simulink model "PWMGenerator"  (R2014a)
settings: Solver=FixedStepDiscrete  StartTime=0.0  StopTime=500000  FixedStep=1  RelTol=1e-3
libraries: hdlsllib x15
settings Model: Creator=rogers.a  LastModifiedBy=rogers.a
settings OptimizationCC: BlockReduction=off  ConditionallyExecuteInputs=off  InlineParams=on
settings DebuggingCC: AlgebraicLoopMsg=error
settings HardwareCC: ProdHWDeviceType=ASIC/FPGA->ASIC/FPGA  ProdEqTarget=off

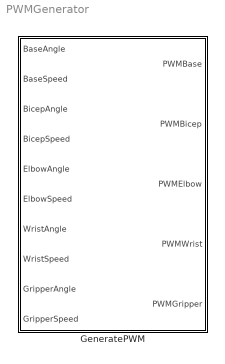
== system PWMGenerator ==
  GeneratePWM : Subsystem  TreatAsAtomicUnit=on

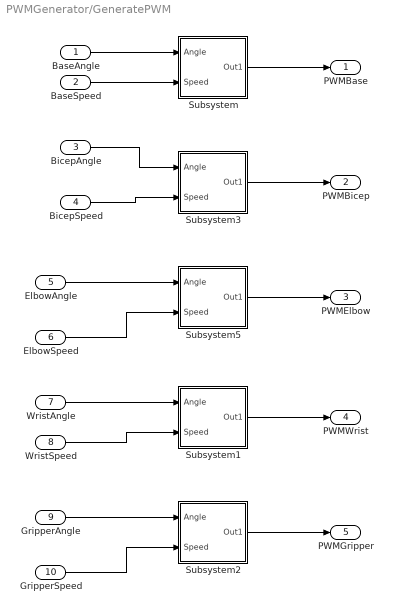
== system PWMGenerator/GeneratePWM ==
  "BaseAngle " : Inport  OutDataTypeStr=int8
  "BaseSpeed " : Inport  Port=2  OutDataTypeStr=int8
  BicepAngle : Inport  Port=3  OutDataTypeStr=int8
  "BicepSpeed " : Inport  Port=4  OutDataTypeStr=int8
  ElbowAngle : Inport  Port=5  OutDataTypeStr=int8
  "ElbowSpeed " : Inport  Port=6  OutDataTypeStr=int8
  WristAngle : Inport  Port=7  OutDataTypeStr=int8
  WristSpeed : Inport  Port=8  OutDataTypeStr=int8
  "GripperAngle " : Inport  Port=9  OutDataTypeStr=int8
  GripperSpeed : Inport  Port=10  OutDataTypeStr=int8
  Subsystem : Subsystem
  Subsystem1 : Subsystem
  Subsystem2 : Subsystem
  Subsystem3 : Subsystem
  Subsystem5 : Subsystem
  PWMBase : Outport
  PWMBicep : Outport  Port=2
  PWMElbow : Outport  Port=3
  PWMWrist : Outport  Port=4
  PWMGripper : Outport  Port=5
  wires:
  Subsystem3/1(Out1) -> PWMBicep/1
  Subsystem5/1(Out1) -> PWMElbow/1
  ElbowAngle/1 -> Subsystem5/1(Angle)
  "ElbowSpeed "/1 -> Subsystem5/2("Speed ")
  Subsystem/1(Out1) -> PWMBase/1
  Subsystem1/1(Out1) -> PWMWrist/1
  WristAngle/1 -> Subsystem1/1(Angle)
  WristSpeed/1 -> Subsystem1/2("Speed ")
  "BaseSpeed "/1 -> Subsystem/2("Speed ")
  "BicepSpeed "/1 -> Subsystem3/2("Speed ")
  "BaseAngle "/1 -> Subsystem/1(Angle)
  BicepAngle/1 -> Subsystem3/1(Angle)
  GripperSpeed/1 -> Subsystem2/2("Speed ")
  "GripperAngle "/1 -> Subsystem2/1(Angle)
  Subsystem2/1(Out1) -> PWMGripper/1

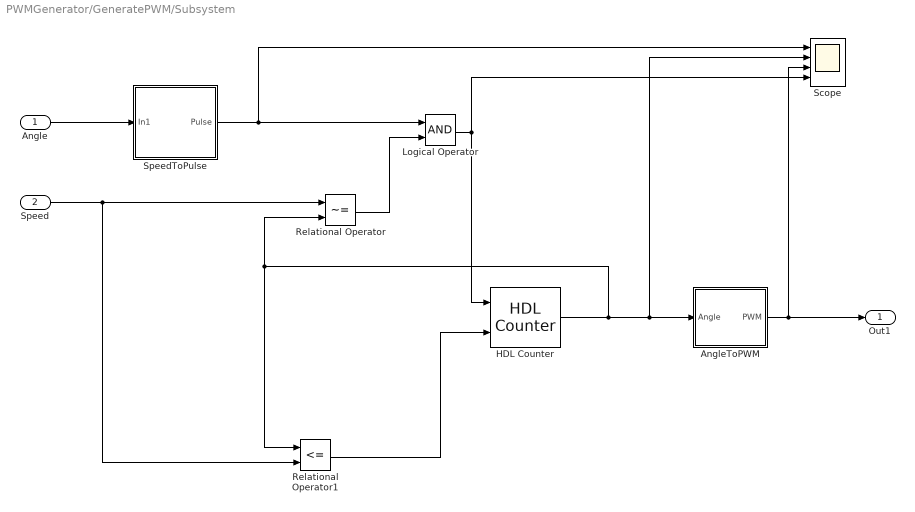
== system PWMGenerator/GeneratePWM/Subsystem ==
  Angle : Inport
  "Speed " : Inport  Port=2
  "AngleToPWM " : Subsystem
  HDL Counter : hdlsllib/HDL Operations/HDL Counter  CountType=Count limited  CountInit=0  CountStep=1  CountMax=180  CountFromType=Specify  CountFrom=0  CountResetPort=off  CountLoadPort=off  CountEnbPort=on  CountDirPort=on  CountDataType=Unsigned  CountWordLen=8  CountFracLen=0  CountSampTime=1
  Logical Operator : Logic  AllPortsSameDT=off  OutDataTypeStr=boolean
  Relational Operator : RelationalOperator  Operator=~=  OutDataTypeStr=boolean
  Relational Operator1 : RelationalOperator  Operator=<=  OutDataTypeStr=boolean
  Scope : Scope  NumInputPorts=4
      settings: YMin=0~0~0~0  YMax=1~300~1~1
  SpeedToPulse : Subsystem
  Out1 : Outport  OutDataTypeStr=boolean
  wires:
  "AngleToPWM "/1("PWM ") -> Scope/3, Out1/1
  HDL Counter/1 -> "AngleToPWM "/1("Angle "), Scope/2, Relational Operator1/1, Relational Operator/2
  Relational Operator1/1 -> HDL Counter/2
  Logical Operator/1 -> Scope/4, HDL Counter/1
  Relational Operator/1 -> Logical Operator/2
  "Speed "/1 -> Relational Operator/1, Relational Operator1/2
  SpeedToPulse/1(Pulse) -> Scope/1, Logical Operator/1
  Angle/1 -> SpeedToPulse/1(In1)

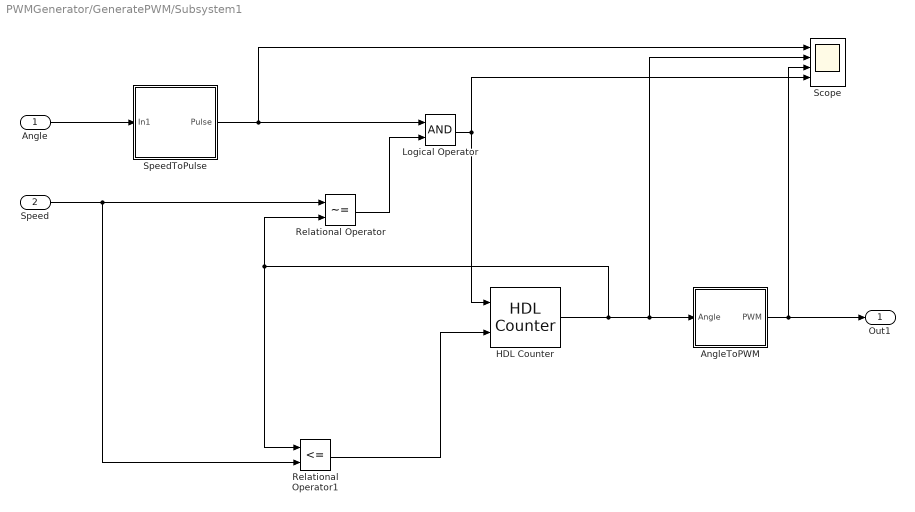
== system PWMGenerator/GeneratePWM/Subsystem1 ==
  Angle : Inport
  "Speed " : Inport  Port=2
  "AngleToPWM " : Subsystem
  HDL Counter : hdlsllib/HDL Operations/HDL Counter  CountType=Count limited  CountInit=0  CountStep=1  CountMax=180  CountFromType=Specify  CountFrom=0  CountResetPort=off  CountLoadPort=off  CountEnbPort=on  CountDirPort=on  CountDataType=Unsigned  CountWordLen=8  CountFracLen=0  CountSampTime=1
  Logical Operator : Logic  AllPortsSameDT=off  OutDataTypeStr=boolean
  Relational Operator : RelationalOperator  Operator=~=  OutDataTypeStr=boolean
  Relational Operator1 : RelationalOperator  Operator=<=  OutDataTypeStr=boolean
  Scope : Scope  NumInputPorts=4
      settings: YMin=0~0~0~0  YMax=1~300~1~1
  SpeedToPulse : Subsystem
  Out1 : Outport  OutDataTypeStr=boolean
  wires:
  "AngleToPWM "/1("PWM ") -> Scope/3, Out1/1
  HDL Counter/1 -> "AngleToPWM "/1("Angle "), Scope/2, Relational Operator1/1, Relational Operator/2
  Relational Operator1/1 -> HDL Counter/2
  Logical Operator/1 -> Scope/4, HDL Counter/1
  Relational Operator/1 -> Logical Operator/2
  "Speed "/1 -> Relational Operator/1, Relational Operator1/2
  SpeedToPulse/1(Pulse) -> Scope/1, Logical Operator/1
  Angle/1 -> SpeedToPulse/1(In1)

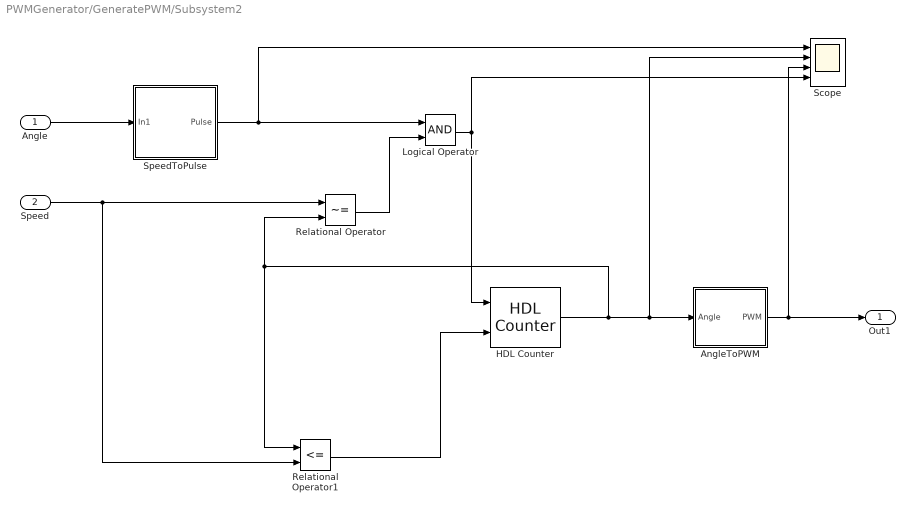
== system PWMGenerator/GeneratePWM/Subsystem2 ==
  Angle : Inport
  "Speed " : Inport  Port=2
  "AngleToPWM " : Subsystem
  HDL Counter : hdlsllib/HDL Operations/HDL Counter  CountType=Count limited  CountInit=0  CountStep=1  CountMax=180  CountFromType=Specify  CountFrom=0  CountResetPort=off  CountLoadPort=off  CountEnbPort=on  CountDirPort=on  CountDataType=Unsigned  CountWordLen=8  CountFracLen=0  CountSampTime=1
  Logical Operator : Logic  AllPortsSameDT=off  OutDataTypeStr=boolean
  Relational Operator : RelationalOperator  Operator=~=  OutDataTypeStr=boolean
  Relational Operator1 : RelationalOperator  Operator=<=  OutDataTypeStr=boolean
  Scope : Scope  NumInputPorts=4
      settings: YMin=0~0~0~0  YMax=1~300~1~1
  SpeedToPulse : Subsystem
  Out1 : Outport  OutDataTypeStr=boolean
  wires:
  "AngleToPWM "/1("PWM ") -> Scope/3, Out1/1
  HDL Counter/1 -> "AngleToPWM "/1("Angle "), Scope/2, Relational Operator1/1, Relational Operator/2
  Relational Operator1/1 -> HDL Counter/2
  Logical Operator/1 -> Scope/4, HDL Counter/1
  Relational Operator/1 -> Logical Operator/2
  "Speed "/1 -> Relational Operator/1, Relational Operator1/2
  SpeedToPulse/1(Pulse) -> Scope/1, Logical Operator/1
  Angle/1 -> SpeedToPulse/1(In1)

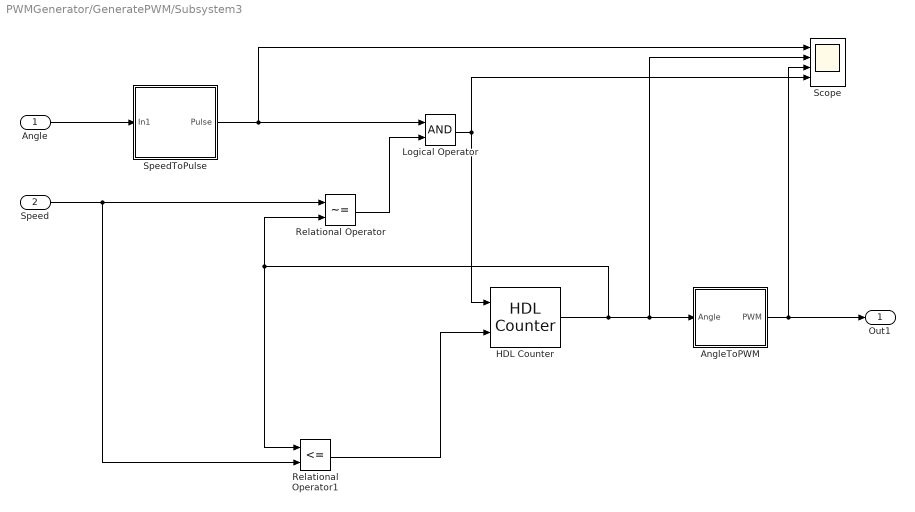
== system PWMGenerator/GeneratePWM/Subsystem3 ==
  Angle : Inport
  "Speed " : Inport  Port=2
  "AngleToPWM " : Subsystem
  HDL Counter : hdlsllib/HDL Operations/HDL Counter  CountType=Count limited  CountInit=0  CountStep=1  CountMax=180  CountFromType=Specify  CountFrom=0  CountResetPort=off  CountLoadPort=off  CountEnbPort=on  CountDirPort=on  CountDataType=Unsigned  CountWordLen=8  CountFracLen=0  CountSampTime=1
  Logical Operator : Logic  AllPortsSameDT=off  OutDataTypeStr=boolean
  Relational Operator : RelationalOperator  Operator=~=  OutDataTypeStr=boolean
  Relational Operator1 : RelationalOperator  Operator=<=  OutDataTypeStr=boolean
  Scope : Scope  NumInputPorts=4
      settings: YMin=0~0~0~0  YMax=1~300~1~1
  SpeedToPulse : Subsystem
  Out1 : Outport  OutDataTypeStr=boolean
  wires:
  "AngleToPWM "/1("PWM ") -> Scope/3, Out1/1
  HDL Counter/1 -> "AngleToPWM "/1("Angle "), Scope/2, Relational Operator1/1, Relational Operator/2
  Relational Operator1/1 -> HDL Counter/2
  Logical Operator/1 -> Scope/4, HDL Counter/1
  Relational Operator/1 -> Logical Operator/2
  "Speed "/1 -> Relational Operator/1, Relational Operator1/2
  SpeedToPulse/1(Pulse) -> Scope/1, Logical Operator/1
  Angle/1 -> SpeedToPulse/1(In1)

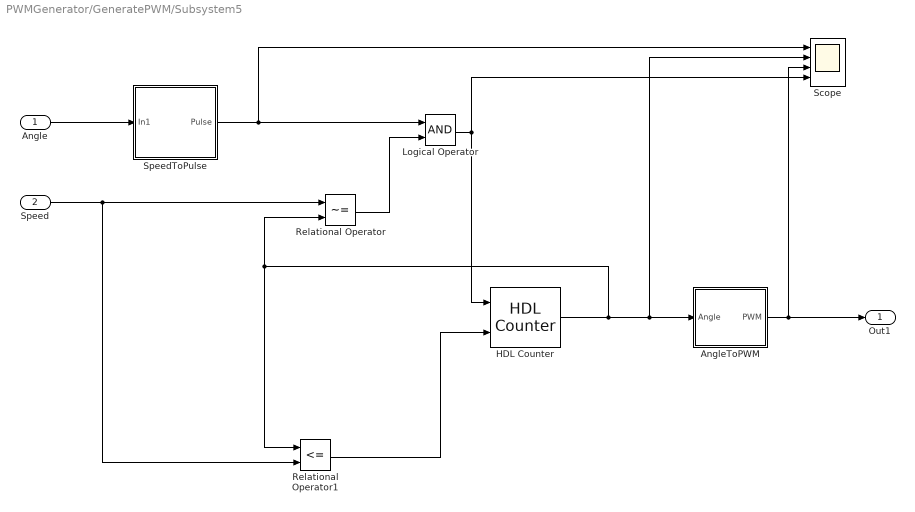
== system PWMGenerator/GeneratePWM/Subsystem5 ==
  Angle : Inport
  "Speed " : Inport  Port=2
  "AngleToPWM " : Subsystem
  HDL Counter : hdlsllib/HDL Operations/HDL Counter  CountType=Count limited  CountInit=0  CountStep=1  CountMax=180  CountFromType=Specify  CountFrom=0  CountResetPort=off  CountLoadPort=off  CountEnbPort=on  CountDirPort=on  CountDataType=Unsigned  CountWordLen=8  CountFracLen=0  CountSampTime=1
  Logical Operator : Logic  AllPortsSameDT=off  OutDataTypeStr=boolean
  Relational Operator : RelationalOperator  Operator=~=  OutDataTypeStr=boolean
  Relational Operator1 : RelationalOperator  Operator=<=  OutDataTypeStr=boolean
  Scope : Scope  NumInputPorts=4
      settings: YMin=0~0~0~0  YMax=1~300~1~1
  SpeedToPulse : Subsystem
  Out1 : Outport  OutDataTypeStr=boolean
  wires:
  "AngleToPWM "/1("PWM ") -> Scope/3, Out1/1
  HDL Counter/1 -> "AngleToPWM "/1("Angle "), Scope/2, Relational Operator1/1, Relational Operator/2
  Relational Operator1/1 -> HDL Counter/2
  Logical Operator/1 -> Scope/4, HDL Counter/1
  Relational Operator/1 -> Logical Operator/2
  "Speed "/1 -> Relational Operator/1, Relational Operator1/2
  SpeedToPulse/1(Pulse) -> Scope/1, Logical Operator/1
  Angle/1 -> SpeedToPulse/1(In1)

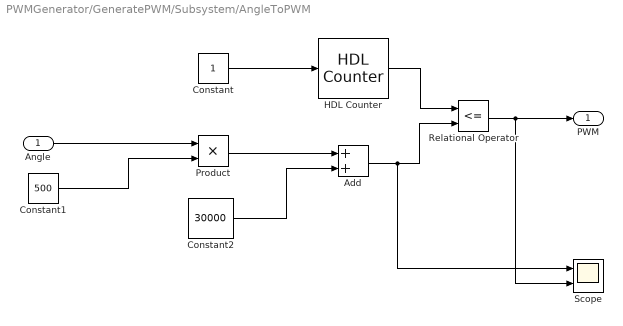
== system PWMGenerator/GeneratePWM/Subsystem/AngleToPWM  ==
  "Angle " : Inport  OutDataTypeStr=uint8
  Add : Sum
  Constant : Constant  OutDataTypeStr=boolean
  Constant1 : Constant  Value=500  OutDataTypeStr=uint32
  Constant2 : Constant  Value=30000  OutDataTypeStr=uint32
  HDL Counter : hdlsllib/HDL Operations/HDL Counter  CountType=Count limited  CountInit=0  CountStep=1  CountMax=1000000  CountFromType=Initial value  CountFrom=0  CountResetPort=off  CountLoadPort=off  CountEnbPort=on  CountDirPort=off  CountDataType=Unsigned  CountWordLen=32  CountFracLen=0  CountSampTime=1
  Product : Product  OutDataTypeStr=Inherit: Inherit via back propagation  SaturateOnIntegerOverflow=on
  Relational Operator : RelationalOperator  Operator=<=  OutDataTypeStr=boolean
  Scope : Scope  NumInputPorts=2
      settings: YMin=45000~-5  YMax=45000~5
  "PWM " : Outport
  wires:
  Add/1 -> Relational Operator/2, Scope/1
  Relational Operator/1 -> "PWM "/1, Scope/2
  "Angle "/1 -> Product/1
  Product/1 -> Add/1
  Constant1/1 -> Product/2
  Constant/1 -> HDL Counter/1
  Constant2/1 -> Add/2
  HDL Counter/1 -> Relational Operator/1

== system PWMGenerator/GeneratePWM/Subsystem/SpeedToPulse ==
  In1 : Inport
  Constant : Constant  Value=50000000  OutDataTypeStr=int32
  Constant1 : Constant  OutDataTypeStr=boolean
  Divide : Product  Inputs=*/  SaturateOnIntegerOverflow=on  RndMeth=Zero
  HDL Counter : hdlsllib/HDL Operations/HDL Counter  CountType=Free running  CountInit=0  CountStep=1  CountMax=10000  CountFromType=Initial value  CountFrom=0  CountResetPort=on  CountLoadPort=off  CountEnbPort=on  CountDirPort=off  CountDataType=Unsigned  CountWordLen=32  CountFracLen=0  CountSampTime=1
  Relational Operator : RelationalOperator  OutDataTypeStr=boolean
  Scope : Scope
  Pulse : Outport
  wires:
  Constant1/1 -> HDL Counter/2
  Relational Operator/1 -> HDL Counter/1, Scope/1, Pulse/1
  In1/1 -> Divide/2
  Divide/1 -> Relational Operator/2
  Constant/1 -> Divide/1
  HDL Counter/1 -> Relational Operator/1

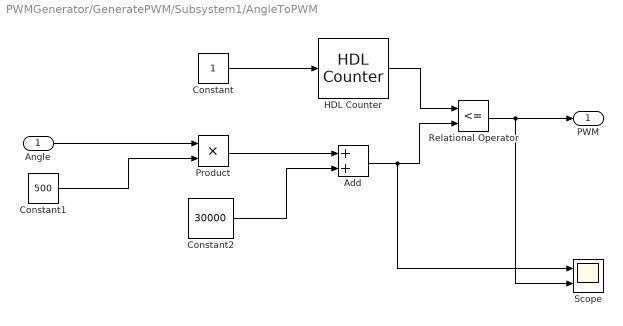
== system PWMGenerator/GeneratePWM/Subsystem1/AngleToPWM  ==
  "Angle " : Inport  OutDataTypeStr=uint8
  Add : Sum
  Constant : Constant  OutDataTypeStr=boolean
  Constant1 : Constant  Value=500  OutDataTypeStr=uint32
  Constant2 : Constant  Value=30000  OutDataTypeStr=uint32
  HDL Counter : hdlsllib/HDL Operations/HDL Counter  CountType=Count limited  CountInit=0  CountStep=1  CountMax=1000000  CountFromType=Initial value  CountFrom=0  CountResetPort=off  CountLoadPort=off  CountEnbPort=on  CountDirPort=off  CountDataType=Unsigned  CountWordLen=32  CountFracLen=0  CountSampTime=1
  Product : Product  OutDataTypeStr=Inherit: Inherit via back propagation  SaturateOnIntegerOverflow=on
  Relational Operator : RelationalOperator  Operator=<=  OutDataTypeStr=boolean
  Scope : Scope  NumInputPorts=2
      settings: YMin=45000~-5  YMax=45000~5
  "PWM " : Outport
  wires:
  Add/1 -> Relational Operator/2, Scope/1
  Relational Operator/1 -> "PWM "/1, Scope/2
  "Angle "/1 -> Product/1
  Product/1 -> Add/1
  Constant1/1 -> Product/2
  Constant/1 -> HDL Counter/1
  Constant2/1 -> Add/2
  HDL Counter/1 -> Relational Operator/1

== system PWMGenerator/GeneratePWM/Subsystem1/SpeedToPulse ==
  In1 : Inport
  Constant : Constant  Value=50000000  OutDataTypeStr=int32
  Constant1 : Constant  OutDataTypeStr=boolean
  Divide : Product  Inputs=*/  SaturateOnIntegerOverflow=on  RndMeth=Zero
  HDL Counter : hdlsllib/HDL Operations/HDL Counter  CountType=Free running  CountInit=0  CountStep=1  CountMax=10000  CountFromType=Initial value  CountFrom=0  CountResetPort=on  CountLoadPort=off  CountEnbPort=on  CountDirPort=off  CountDataType=Unsigned  CountWordLen=32  CountFracLen=0  CountSampTime=1
  Relational Operator : RelationalOperator  OutDataTypeStr=boolean
  Scope : Scope
  Pulse : Outport
  wires:
  Constant1/1 -> HDL Counter/2
  Relational Operator/1 -> HDL Counter/1, Scope/1, Pulse/1
  In1/1 -> Divide/2
  Divide/1 -> Relational Operator/2
  Constant/1 -> Divide/1
  HDL Counter/1 -> Relational Operator/1

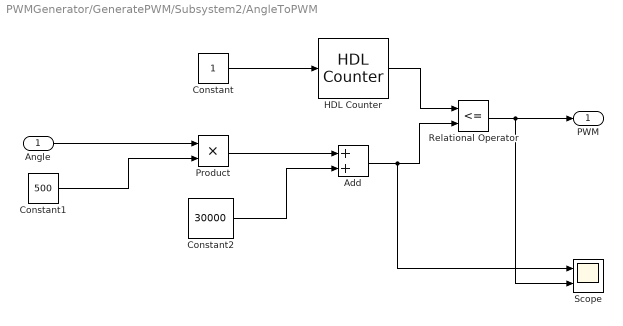
== system PWMGenerator/GeneratePWM/Subsystem2/AngleToPWM  ==
  "Angle " : Inport  OutDataTypeStr=uint8
  Add : Sum
  Constant : Constant  OutDataTypeStr=boolean
  Constant1 : Constant  Value=500  OutDataTypeStr=uint32
  Constant2 : Constant  Value=30000  OutDataTypeStr=uint32
  HDL Counter : hdlsllib/HDL Operations/HDL Counter  CountType=Count limited  CountInit=0  CountStep=1  CountMax=1000000  CountFromType=Initial value  CountFrom=0  CountResetPort=off  CountLoadPort=off  CountEnbPort=on  CountDirPort=off  CountDataType=Unsigned  CountWordLen=32  CountFracLen=0  CountSampTime=1
  Product : Product  OutDataTypeStr=Inherit: Inherit via back propagation  SaturateOnIntegerOverflow=on
  Relational Operator : RelationalOperator  Operator=<=  OutDataTypeStr=boolean
  Scope : Scope  NumInputPorts=2
      settings: YMin=45000~-5  YMax=45000~5
  "PWM " : Outport
  wires:
  Add/1 -> Relational Operator/2, Scope/1
  Relational Operator/1 -> "PWM "/1, Scope/2
  "Angle "/1 -> Product/1
  Product/1 -> Add/1
  Constant1/1 -> Product/2
  Constant/1 -> HDL Counter/1
  Constant2/1 -> Add/2
  HDL Counter/1 -> Relational Operator/1

== system PWMGenerator/GeneratePWM/Subsystem2/SpeedToPulse ==
  In1 : Inport
  Constant : Constant  Value=50000000  OutDataTypeStr=int32
  Constant1 : Constant  OutDataTypeStr=boolean
  Divide : Product  Inputs=*/  SaturateOnIntegerOverflow=on  RndMeth=Zero
  HDL Counter : hdlsllib/HDL Operations/HDL Counter  CountType=Free running  CountInit=0  CountStep=1  CountMax=10000  CountFromType=Initial value  CountFrom=0  CountResetPort=on  CountLoadPort=off  CountEnbPort=on  CountDirPort=off  CountDataType=Unsigned  CountWordLen=32  CountFracLen=0  CountSampTime=1
  Relational Operator : RelationalOperator  OutDataTypeStr=boolean
  Scope : Scope
  Pulse : Outport
  wires:
  Constant1/1 -> HDL Counter/2
  Relational Operator/1 -> HDL Counter/1, Scope/1, Pulse/1
  In1/1 -> Divide/2
  Divide/1 -> Relational Operator/2
  Constant/1 -> Divide/1
  HDL Counter/1 -> Relational Operator/1

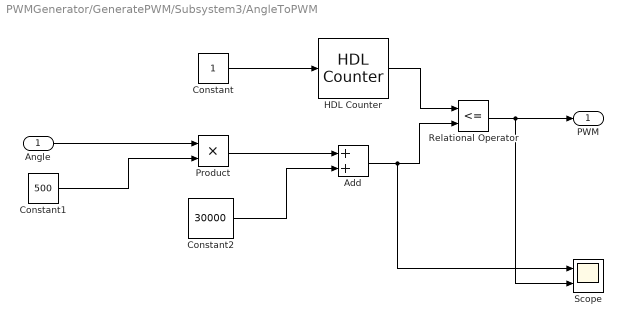
== system PWMGenerator/GeneratePWM/Subsystem3/AngleToPWM  ==
  "Angle " : Inport  OutDataTypeStr=uint8
  Add : Sum
  Constant : Constant  OutDataTypeStr=boolean
  Constant1 : Constant  Value=500  OutDataTypeStr=uint32
  Constant2 : Constant  Value=30000  OutDataTypeStr=uint32
  HDL Counter : hdlsllib/HDL Operations/HDL Counter  CountType=Count limited  CountInit=0  CountStep=1  CountMax=1000000  CountFromType=Initial value  CountFrom=0  CountResetPort=off  CountLoadPort=off  CountEnbPort=on  CountDirPort=off  CountDataType=Unsigned  CountWordLen=32  CountFracLen=0  CountSampTime=1
  Product : Product  OutDataTypeStr=Inherit: Inherit via back propagation  SaturateOnIntegerOverflow=on
  Relational Operator : RelationalOperator  Operator=<=  OutDataTypeStr=boolean
  Scope : Scope  NumInputPorts=2
      settings: YMin=45000~-5  YMax=45000~5
  "PWM " : Outport
  wires:
  Add/1 -> Relational Operator/2, Scope/1
  Relational Operator/1 -> "PWM "/1, Scope/2
  "Angle "/1 -> Product/1
  Product/1 -> Add/1
  Constant1/1 -> Product/2
  Constant/1 -> HDL Counter/1
  Constant2/1 -> Add/2
  HDL Counter/1 -> Relational Operator/1

== system PWMGenerator/GeneratePWM/Subsystem3/SpeedToPulse ==
  In1 : Inport
  Constant : Constant  Value=50000000  OutDataTypeStr=int32
  Constant1 : Constant  OutDataTypeStr=boolean
  Divide : Product  Inputs=*/  SaturateOnIntegerOverflow=on  RndMeth=Zero
  HDL Counter : hdlsllib/HDL Operations/HDL Counter  CountType=Free running  CountInit=0  CountStep=1  CountMax=10000  CountFromType=Initial value  CountFrom=0  CountResetPort=on  CountLoadPort=off  CountEnbPort=on  CountDirPort=off  CountDataType=Unsigned  CountWordLen=32  CountFracLen=0  CountSampTime=1
  Relational Operator : RelationalOperator  OutDataTypeStr=boolean
  Scope : Scope
  Pulse : Outport
  wires:
  Constant1/1 -> HDL Counter/2
  Relational Operator/1 -> HDL Counter/1, Scope/1, Pulse/1
  In1/1 -> Divide/2
  Divide/1 -> Relational Operator/2
  Constant/1 -> Divide/1
  HDL Counter/1 -> Relational Operator/1

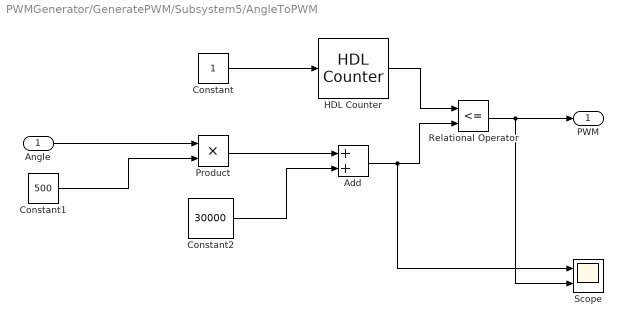
== system PWMGenerator/GeneratePWM/Subsystem5/AngleToPWM  ==
  "Angle " : Inport  OutDataTypeStr=uint8
  Add : Sum
  Constant : Constant  OutDataTypeStr=boolean
  Constant1 : Constant  Value=500  OutDataTypeStr=uint32
  Constant2 : Constant  Value=30000  OutDataTypeStr=uint32
  HDL Counter : hdlsllib/HDL Operations/HDL Counter  CountType=Count limited  CountInit=0  CountStep=1  CountMax=1000000  CountFromType=Initial value  CountFrom=0  CountResetPort=off  CountLoadPort=off  CountEnbPort=on  CountDirPort=off  CountDataType=Unsigned  CountWordLen=32  CountFracLen=0  CountSampTime=1
  Product : Product  OutDataTypeStr=Inherit: Inherit via back propagation  SaturateOnIntegerOverflow=on
  Relational Operator : RelationalOperator  Operator=<=  OutDataTypeStr=boolean
  Scope : Scope  NumInputPorts=2
      settings: YMin=45000~-5  YMax=45000~5
  "PWM " : Outport
  wires:
  Add/1 -> Relational Operator/2, Scope/1
  Relational Operator/1 -> "PWM "/1, Scope/2
  "Angle "/1 -> Product/1
  Product/1 -> Add/1
  Constant1/1 -> Product/2
  Constant/1 -> HDL Counter/1
  Constant2/1 -> Add/2
  HDL Counter/1 -> Relational Operator/1

== system PWMGenerator/GeneratePWM/Subsystem5/SpeedToPulse ==
  In1 : Inport
  Constant : Constant  Value=50000000  OutDataTypeStr=int32
  Constant1 : Constant  OutDataTypeStr=boolean
  Divide : Product  Inputs=*/  SaturateOnIntegerOverflow=on  RndMeth=Zero
  HDL Counter : hdlsllib/HDL Operations/HDL Counter  CountType=Free running  CountInit=0  CountStep=1  CountMax=10000  CountFromType=Initial value  CountFrom=0  CountResetPort=on  CountLoadPort=off  CountEnbPort=on  CountDirPort=off  CountDataType=Unsigned  CountWordLen=32  CountFracLen=0  CountSampTime=1
  Relational Operator : RelationalOperator  OutDataTypeStr=boolean
  Scope : Scope
  Pulse : Outport
  wires:
  Constant1/1 -> HDL Counter/2
  Relational Operator/1 -> HDL Counter/1, Scope/1, Pulse/1
  In1/1 -> Divide/2
  Divide/1 -> Relational Operator/2
  Constant/1 -> Divide/1
  HDL Counter/1 -> Relational Operator/1
